simulink model "tarefa_6_5"  (R2023b)
settings: Solver=VariableStepAuto  StartTime=0.0  StopTime=t  FixedStep=passo  RelTol=1e-3
InitFcn:
  | t = 1.6;
  | 
  | % Parametros da rede
  | Vabc = 380;
  | Vrede = Vabc*sqrt(2)/sqrt(3);
  | Frede = 60;
  | Vdc = 700;
  | fsw = 6e3;
  | 
  | % Parametros Filtro
  | Lg = 406.3e-6;
  | Cf = 31.1744e-6;
  | Rd = 1;
  | Lf = Lg;
  | L = Lg+Lf;
  | R = 2*pi*Frede*L/40;
  | 
  | % Parametros PLL
  | Winit = 2*pi*60;
  | ksi_srf = 1/sqrt(2);
  | wn_srf = 20*2*pi;
  | Vg = Vrede;
  | Kp_pll = 2*wn_srf*ksi_srf/Vg;
  | Ki_pll = (wn_srf^2)/Vg;
  | 
  | % Malha Interna PI
  | fcd = fsw/20;
  | Kp_int_pi = 2*pi*fcd*L;
  | Ki_int = 2*pi*fcd*R;
  | wnL = 2*pi*Frede*L;
  | 
  | 
  | % Aula hoje
  | %Capacitor barramento
  | P = 20e3;
  | c_bar = 4e-3;
  | 
  | %controle do eixo de potencia reativa
  | fc1 = fcd/5;
  | fc2 = fc1/5;
  | kp_rea = 2*pi*fc2/(-(2*pi*fc1-2*pi*fc2)*1.5*sqrt(2)*Vrede/sqrt(3));
  | ki_rea = 2*pi*fc1*kp_rea;
  | 
  | % Tensão do barramento
  | 
  | G = 1.5*Vabc*sqrt(2/3)/Vdc;
  | kp_bar = 2*pi* (fc1 + fc2)*c_bar/G;
  | ki_bar = 4*pi^2* fc1*fc2*c_bar/G;
  | 
  | kp_bar_2 = c_bar*pi*(fc1 + fc2);
  | ki_bar_2 = (2*pi^2)*c_bar*(fc1 + fc2);
undefined symbols (not defined in the file): plecs
settings Model: PacingRate=0.020000  Creator=unknow  LastModifiedBy=unknow

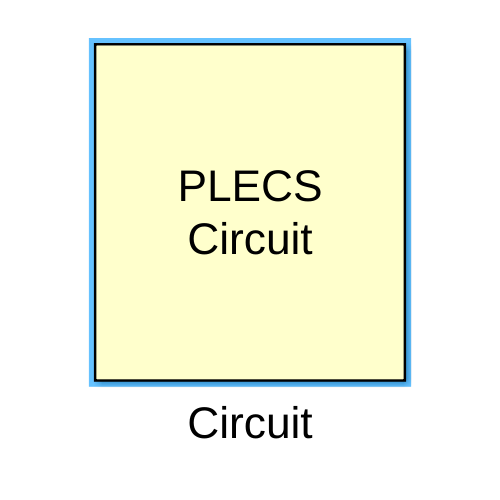
[thumbnail: Simulink's stored preview of the top-level diagram]
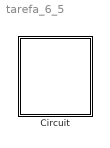
== system tarefa_6_5 ==
  Circuit : Subsystem  LoadFcn=plecs('sl', 200);  InitFcn=plecs('sl', 214);  StartFcn=plecs('sl', 208);  StopFcn=plecs('sl', 209);  mask(PlecsCircuit){PLECSData=<binary blob, 16092 chars, not shown>}
      mask prompts: PLECSData "PLECS Data (Do not delete or modify!)"
      mask init:
      | % PLACE CUSTOM INITIALIZATIONS ABOVE
      | % DO NOT REMOVE
      | plecs('sl', 215);
      | % DO NOT REMOVE
      settings: CopyFcn=plecs('sl', 203);  DeleteFcn=plecs('sl', 205);  UndoDeleteFcn=plecs('sl', 206);  PreSaveFcn=plecs('sl', 211);  PostSaveFcn=plecs('sl', 201);  NameChangeFcn=plecs('sl', 210);  DestroyFcn=plecs('sl', 207);  PreCopyFcn=plecs('sl', 216);  OpenFcn=plecs('sl', 202);  ErrorFcn=plerrorfcn
      mask Help: eval('plecs(''help'', ''qthelp:///creatingacircuit.html'')')
      mask Display: disp('PLECS\nCircuit')

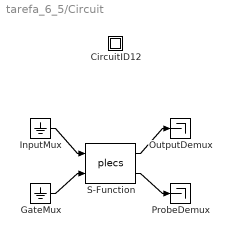
== system tarefa_6_5/Circuit ==
  " CircuitID12 " : Subsystem
  " GateMux " : Ground
  " InputMux " : Ground
  " OutputDemux " : Terminator
  " ProbeDemux " : Terminator
  " S-Function " : S-Function  FunctionName=plecs  SFunctionDeploymentMode=off  EnableBusSupport=off
  wires:
  " InputMux "/1 -> " S-Function "/1
  " GateMux "/1 -> " S-Function "/2
  " S-Function "/1 -> " OutputDemux "/1
  " S-Function "/2 -> " ProbeDemux "/1

== system tarefa_6_5/Circuit/ CircuitID12  ==
